simulink model "Solucion_ecuacion_diferencial_Matlab"  (R2022a)
settings: Solver=VariableStepAuto  StartTime=0.0  StopTime=10.0  RelTol=1e-3
settings Model: Creator=rafae  LastModifiedBy=rafae

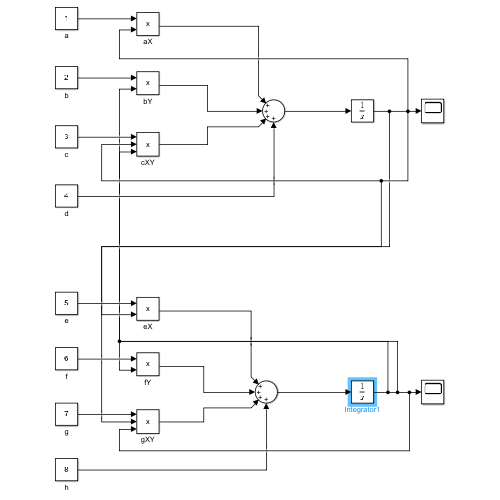
[thumbnail: Simulink's stored preview of the top-level diagram]
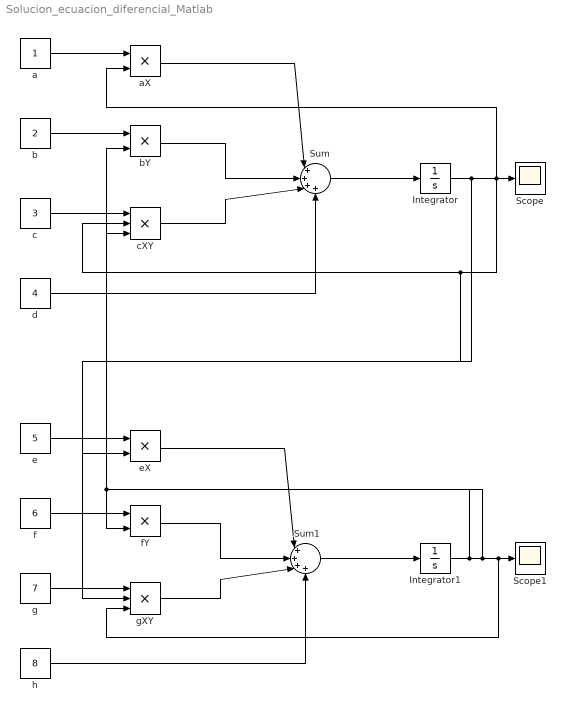
== system Solucion_ecuacion_diferencial_Matlab ==
  Integrator : Integrator  InitialCondition=10
  Integrator1 : Integrator  InitialCondition=1
  Scope : Scope
  Scope1 : Scope
  Sum : Sum  Inputs=|++++
  Sum1 : Sum  Inputs=|++++
  a : Constant
  aX : Product
  b : Constant  Value=2
  bY : Product
  c : Constant  Value=3
  cXY : Product  Inputs=3
  d : Constant  Value=4
  e : Constant  Value=5
  eX : Product
  f : Constant  Value=6
  fY : Product
  g : Constant  Value=7
  gXY : Product  Inputs=3
  h : Constant  Value=8
  wires:
  g/1 -> gXY/1
  e/1 -> eX/1
  f/1 -> fY/1
  c/1 -> cXY/1
  b/1 -> bY/1
  a/1 -> aX/1
  aX/1 -> Sum/1
  bY/1 -> Sum/2
  cXY/1 -> Sum/3
  d/1 -> Sum/4
  eX/1 -> Sum1/1
  fY/1 -> Sum1/2
  gXY/1 -> Sum1/3
  h/1 -> Sum1/4
  Sum/1 -> Integrator/1
  Sum1/1 -> Integrator1/1
  Integrator/1 -> gXY/2, eX/2, cXY/2, aX/2, Scope/1
  Integrator1/1 -> cXY/3, fY/2, bY/2, gXY/3, Scope1/1
